simulink model "SIMULACIO_SUMA_ENTRADES_V2"  (R2020b)
settings: Solver=VariableStepAuto  StartTime=0.0  StopTime=200  RelTol=1e-3
values from neighbouring files (symbols this model uses):
  Guany = 0.97    [valors_model_v2.m]
  k = 1/1000000    (= 1e-06)    [valors_model_v2.m]
  P = g*d*h*n    (= 104182.2)    [valors_model_v2.m]
  R = -0.05    [valors_model_v2.m]
  tau = 0.010    (= 0.01)    [valors_model_v2.m]
libraries: simulink x3
settings Model: Creator=34691  LastModifiedBy=34691

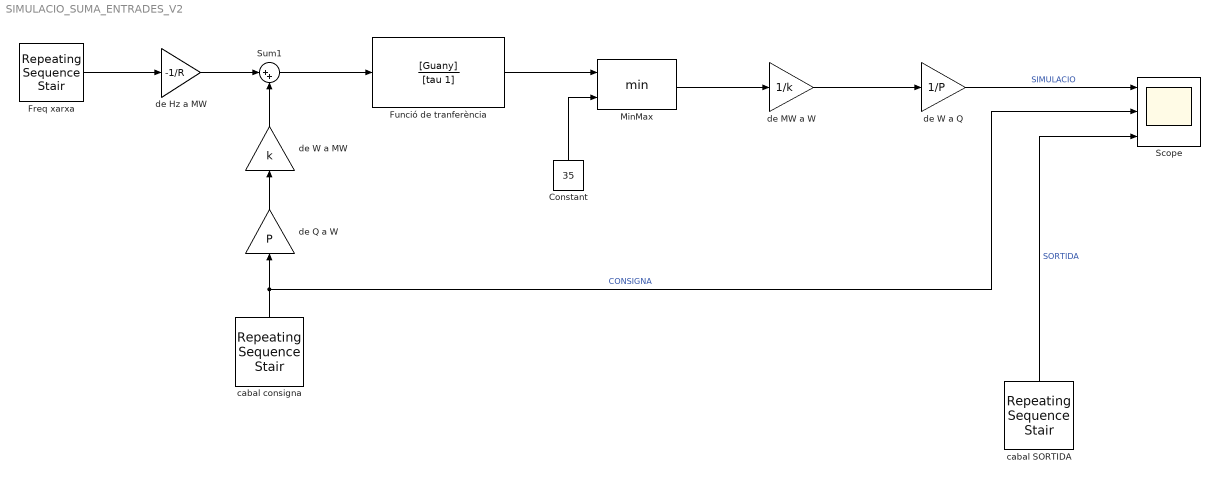
== system SIMULACIO_SUMA_ENTRADES_V2 ==
  Constant : Constant  Value=35
  Freq xarxa : simulink/Sources/Repeating Sequence Stair  OutValues=incr_freq  tsamp=0.5  OutMin=[]  OutMax=[]  OutDataTypeStr=double  OutputDataTypeScalingMode=double  OutDataType=fixdt(0,8)  ConRadixGroup=Best Precision: Vector-wise  OutScaling=2^-12
  Funció de tranferència : TransferFcn  Numerator=[Guany]  Denominator=[tau 1]
  MinMax : MinMax  Inputs=2
  Scope : Scope  NumInputPorts=3
  Sum1 : Sum  Inputs=|++
  cabal SORTIDA : simulink/Sources/Repeating Sequence Stair  OutValues=cabal_sortida  tsamp=0.1  OutMin=[]  OutMax=[]  OutDataTypeStr=double  OutputDataTypeScalingMode=double  OutDataType=fixdt(0,8)  ConRadixGroup=Best Precision: Vector-wise  OutScaling=2^-12
  cabal consigna : simulink/Sources/Repeating Sequence Stair  OutValues=cabal  tsamp=0.1  OutMin=[]  OutMax=[]  OutDataTypeStr=double  OutputDataTypeScalingMode=double  OutDataType=fixdt(0,8)  ConRadixGroup=Best Precision: Vector-wise  OutScaling=2^-12
  de Hz a MW : Gain  Gain=-1/R
  de MW a W : Gain  Gain=1/k
  de Q a W : Gain  Gain=P
  de W a MW : Gain  Gain=k
  de W a Q : Gain  Gain=1/P
  wires:
  Sum1/1 -> Funció de tranferència/1
  Freq xarxa/1 -> de Hz a MW/1
  de Hz a MW/1 -> Sum1/1
  cabal consigna/1 -> de Q a W/1, Scope/2  "CONSIGNA"
  de Q a W/1 -> de W a MW/1
  de W a MW/1 -> Sum1/2
  Funció de tranferència/1 -> MinMax/1
  Constant/1 -> MinMax/2
  MinMax/1 -> de MW a W/1
  de MW a W/1 -> de W a Q/1
  de W a Q/1 -> Scope/1  "SIMULACIO"
  cabal SORTIDA/1 -> Scope/3  "SORTIDA"
